simulink model "Lab3Pre"  (R2015b)
settings: Solver=ode3  StartTime=0.0  StopTime=5  FixedStep=0.01  RelTol=1e-3
undefined symbols (not defined in the file): K
settings Model: Creator=FANUC  LastModifiedBy=FANUC
settings DataIOCC: LimitDataPoints=off  SaveFormat=Array  TimeSaveName=t  OutputSaveName=x

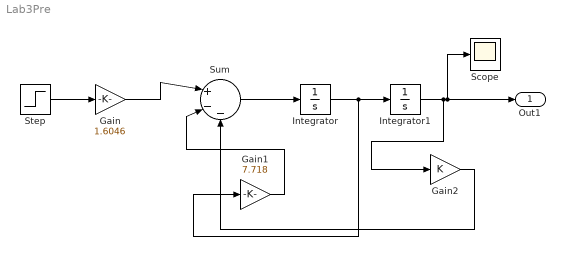
== system Lab3Pre ==
  Gain : Gain  Gain=1.6046
  Gain1 : Gain  Gain=7.718
  Gain2 : Gain  Gain=K
  Integrator : Integrator
  Integrator1 : Integrator
  Scope : Scope
  Step : Step  Time=0  SampleTime=0
  Sum : Sum  Inputs=|+--
  Out1 : Outport
  wires:
  Step/1 -> Gain/1
  Gain/1 -> Sum/1
  Sum/1 -> Integrator/1
  Integrator/1 -> Gain1/1, Integrator1/1
  Gain1/1 -> Sum/2
  Integrator1/1 -> Gain2/1, Out1/1, Scope/1
  Gain2/1 -> Sum/3
